simulink model "govno1"  (R2019b)
settings: Solver=ode45  StartTime=0.0  StopTime=80  RelTol=1e-3  EnableMultiTasking=on
libraries: simulink x3
settings Model: Creator=Lazaros  LastModifiedBy=kWX1197707
settings DataIOCC: SaveFormat=Array  ReturnWorkspaceOutputs=off  Refine=4
settings OptimizationCC: LifeSpan=inf
settings DebuggingCC: UnderspecifiedInitializationDetection=Classic  MergeDetectMultiDrivingBlocksExec=none  SolverPrmCheckMsg=warning  StateNameClashWarn=warning  SFUnexpectedBacktrackingDiag=warning  SFNoUnconditionalDefaultTransitionDiag=warning  SFExecutionAtInitializationDiag=none  ArithmeticOperatorsInVariantConditions=warning
settings HardwareCC: ProdBitPerPointer=32  ProdBitPerSizeT=32  ProdBitPerPtrDiffT=32  ProdLargestAtomicFloat=None  ProdIntDivRoundTo=Undefined  ProdEndianess=Unspecified  ProdWordSize=32  ProdHWDeviceType=32-bit Generic
settings ModelReferenceCC: PropagateSignalLabelsOutOfModel=off
settings SFSimCC: SimUseLocalCustomCode=off  CustomCodeUndefinedFunction=UseInterfaceOnly
settings RTWCC: RTWUseLocalCustomCode=off
settings CodeAppCC: StateflowObjectComments=on
settings GRTTargetCC: TargetLangStandard=C89/C90 (ANSI)  GeneratePreprocessorConditionals=Disable all
settings ConfigComp: CovMetricSettings=dw  CovHtmlReporting=on  CovSaveCumulativeToWorkspaceVar=on  CovSaveSingleToWorkspaceVar=on  CovExternalEMLEnable=off

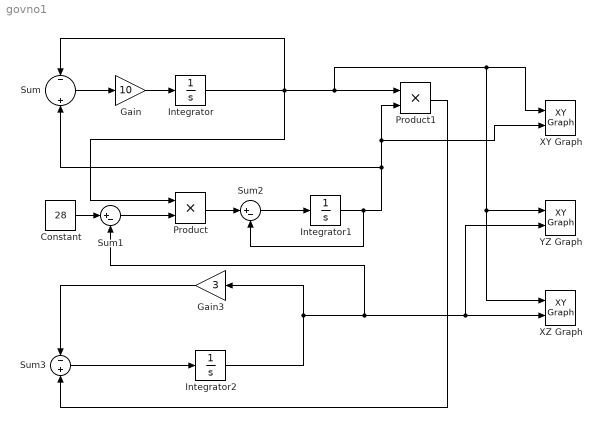
== system govno1 ==
  Constant : Constant  Value=28
  Gain : Gain  Gain=10
  Gain3 : Gain  Gain=3
  Integrator : Integrator  InitialCondition=5
  Integrator1 : Integrator  InitialCondition=5
  Integrator2 : Integrator  InitialCondition=5
  Product : Product
  Product1 : Product
  Sum : Sum  Inputs=-|||+
  Sum1 : Sum  Inputs=|+-
  Sum2 : Sum  Inputs=|+-
  Sum3 : Sum  Inputs=-+
  XY Graph : simulink/Sinks/XY Graph  xmin=-20  xmax=20  ymin=-30  ymax=30  st=-1
  XZ Graph : simulink/Sinks/XY Graph  xmin=-20  xmax=20  ymin=-0  ymax=60  st=-1
  YZ Graph : simulink/Sinks/XY Graph  xmin=-20  xmax=20  ymin=0  ymax=60  st=-1
  wires:
  Integrator/1 -> XZ Graph/1, YZ Graph/1, XY Graph/1, Product1/1, Product/1, Sum/1
  Sum/1 -> Gain/1
  Gain/1 -> Integrator/1
  Integrator1/1 -> Sum2/2, XY Graph/2, Product1/2, Sum/2
  Integrator2/1 -> Gain3/1, XZ Graph/2, YZ Graph/2, Sum1/2
  Sum1/1 -> Product/2
  Product/1 -> Sum2/1
  Sum2/1 -> Integrator1/1
  Sum3/1 -> Integrator2/1
  Gain3/1 -> Sum3/1
  Product1/1 -> Sum3/2
  Constant/1 -> Sum1/1
